simulink model "longmendiao"  (R2023b)
settings: Solver=FixedStepAuto  StartTime=0.0  StopTime=10.0  FixedStep=0.01  RelTol=1e-3
settings Model: Creator=asus  LastModifiedBy=asus

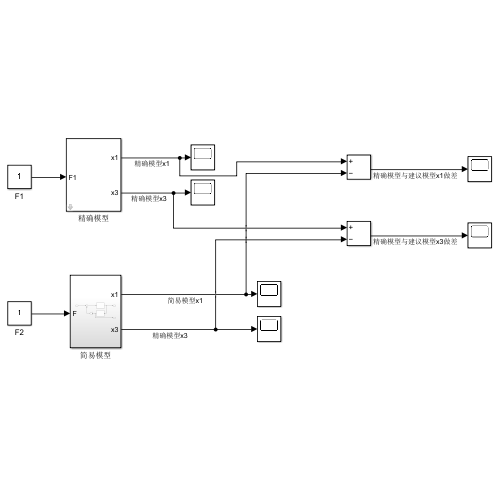
[thumbnail: Simulink's stored preview of the top-level diagram]
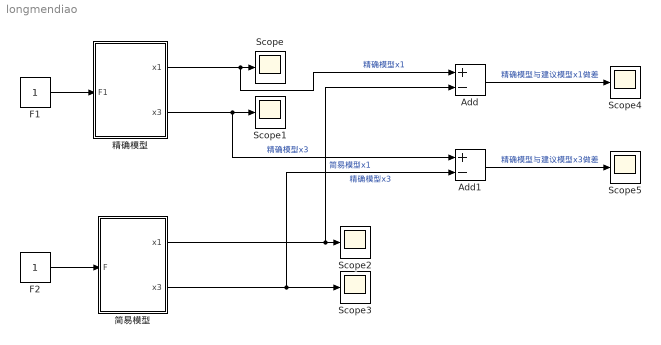
== system longmendiao ==
  Add : Sum  Inputs=+-
  Add1 : Sum  Inputs=+-
  F1 : Constant
  F2 : Constant
  Scope{,1..5} (6 alike) : Scope
  简易模型 : Subsystem
  精确模型 : Subsystem  mask{m0=50, m=5, l=1, D=0, g=9.8, eta=0}
      mask DialogControl ParameterGroupVar Prompt: 参数
  wires:
  F1/1 -> 精确模型/1(F1)
  精确模型/1(x1) -> Add/1, Scope/1  "精确模型x1"
  精确模型/2(x3) -> Add1/1, Scope1/1  "精确模型x3"
  F2/1 -> 简易模型/1(F)
  简易模型/1(x1) -> Add/2, Scope2/1  "简易模型x1"
  简易模型/2(x3) -> Add1/2, Scope3/1  "精确模型x3"
  Add/1 -> Scope4/1  "精确模型与建议模型x1做差"
  Add1/1 -> Scope5/1  "精确模型与建议模型x3做差"

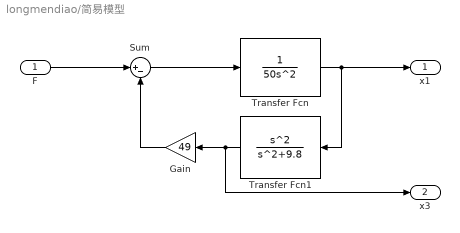
== system longmendiao/简易模型 ==
  F : Inport
  Gain : Gain  Gain=49
  Sum : Sum  Inputs=|+-
  Transfer Fcn : TransferFcn  Denominator=[50 0 0]
  Transfer Fcn1 : TransferFcn  Numerator=[1 0 0]  Denominator=[1 0 9.8]
  x1 : Outport
  x3 : Outport  Port=2
  wires:
  F/1 -> Sum/1
  Transfer Fcn1/1 -> x3/1, Gain/1
  Transfer Fcn/1 -> x1/1, Transfer Fcn1/1
  Sum/1 -> Transfer Fcn/1
  Gain/1 -> Sum/2

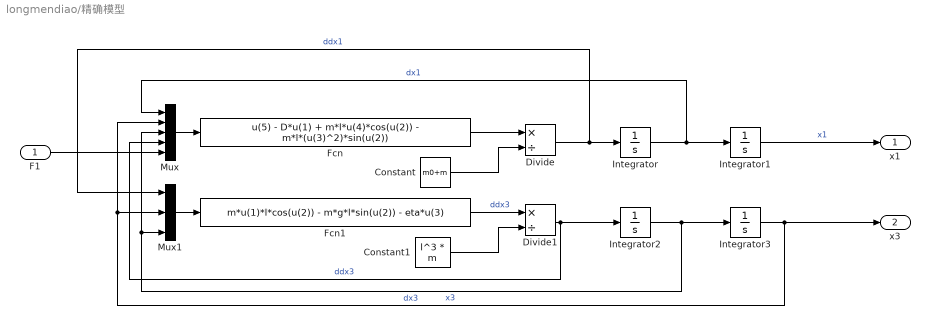
== system longmendiao/精确模型 ==
  F1 : Inport
  Constant : Constant  Value=m0+m
  Constant1 : Constant  Value=l^3 * m
  Divide : Product  Inputs=*/
  Divide1 : Product  Inputs=*/
  Fcn : Fcn  Expr=u(5) - D*u(1) + m*l*u(4)*cos(u(2)) - m*l*(u(3)^2)*sin(u(2))
  Fcn1 : Fcn  Expr=m*u(1)*l*cos(u(2)) - m*g*l*sin(u(2)) - eta*u(3)
  Integrator{,1..3} (4 alike) : Integrator
  Mux : Mux  Inputs=5
  Mux1 : Mux  Inputs=3
  x1 : Outport
  x3 : Outport  Port=2
  wires:
  Integrator/1 -> Mux/1, Integrator1/1  "dx1"
  Divide/1 -> Mux1/1, Integrator/1  "ddx1"
  Fcn/1 -> Divide/1
  Integrator3/1 -> x3/1, Mux1/2, Mux/2  "x3"
  Mux/1 -> Fcn/1
  Divide1/1 -> Mux/4, Integrator2/1  "ddx3"
  Integrator2/1 -> Mux/3, Mux1/3, Integrator3/1  "dx3"
  Constant1/1 -> Divide1/2
  Fcn1/1 -> Divide1/1  "ddx3"
  Constant/1 -> Divide/2
  Mux1/1 -> Fcn1/1
  Integrator1/1 -> x1/1  "x1"
  F1/1 -> Mux/5
